simulink model "BlockTest"  (R2017b)
settings: Solver=FixedStepAuto  StartTime=0.0  StopTime=inf  FixedStep=.005  RelTol=1e-3  EnableMultiTasking=on
libraries: arduinolib x2, RASPlib x1, simulink x1
settings Model: SimulationMode=external  ExtModeTrigDuration=2  Creator=nguye  LastModifiedBy=nguye
settings OptimizationCC: PassReuseOutputArgsAs=Individual arguments  MaxStackSize=64
settings DebuggingCC: ParameterTunabilityLossMsg=error
settings HardwareCC: ProdBitPerInt=16  ProdBitPerPointer=16  ProdBitPerSizeT=16  ProdBitPerPtrDiffT=16  ProdLargestAtomicFloat=None  ProdWordSize=8  ProdHWDeviceType=Atmel->AVR
settings SFSimCC: MATLABDynamicMemAlloc=off
settings RTWCC: SystemTargetFile=ert.tlc  HardwareBoard=Arduino Mega 2560  TLCOptions=-aInlineSetEventsForThisBaseRateFcn=TLC_FALSE -aSuppressMultiTaskScheduler=TLC_FALSE -aRateBasedStepFcn=1  TemplateMakefile=ert_default_tmf  GenerateReport=on  Toolchain=Arduino AVR  BuildConfiguration=Faster Runs  IncludeHyperlinkInReport=on  LaunchReport=on  GenerateTraceInfo=on  GenerateTraceReport=on  GenerateTraceReportSl=on  GenerateTraceReportSf=on  GenerateTraceReportEml=on
settings CodeAppCC: ForceParamTrailComments=on  IgnoreCustomStorageClasses=off  OperatorAnnotations=on  SimulinkDataObjDesc=on  SFDataObjDesc=on  InsertBlockDesc=on
settings ERTTargetCC: SupportContinuousTime=on  SupportVariableSizeSignals=on  ExtMode=on  ExtModeMexArgs='127.0.0.1' 0 17725

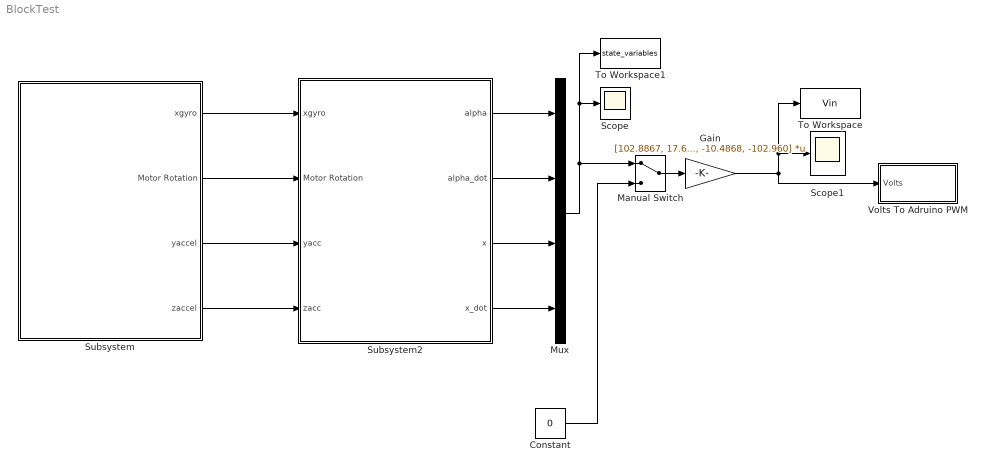
== system BlockTest ==
  Constant : Constant  Value=0
  Gain : Gain  Gain=[102.8867, 17.6796, -10.4868, -102.960]  Multiplication=Matrix(K*u)
  Manual Switch : ManualSwitch
  Mux : Mux
  Scope : Scope
  Scope1 : Scope
  Subsystem : Subsystem
  Subsystem2 : Subsystem
  To Workspace : ToWorkspace  VariableName=Vin  SaveFormat=Timeseries  SampleTime=-1
  To Workspace1 : ToWorkspace  VariableName=state_variables  SampleTime=-1
  Volts To Adruino PWM : Subsystem
  wires:
  Subsystem/1(xgyro) -> Subsystem2/1(xgyro)
  Subsystem/2(Motor Rotation) -> Subsystem2/2(Motor Rotation)
  Mux/1 -> To Workspace1/1, Scope/1, Manual Switch/1
  Manual Switch/1 -> Gain/1
  Constant/1 -> Manual Switch/2
  Gain/1 -> Volts To Adruino PWM/1(Volts), To Workspace/1, Scope1/1
  Subsystem/3(yaccel) -> Subsystem2/3(yacc)
  Subsystem/4(zaccel) -> Subsystem2/4(zacc)
  Subsystem2/4(x_dot) -> Mux/4
  Subsystem2/3(x) -> Mux/3
  Subsystem2/2(alpha_dot) -> Mux/2
  Subsystem2/1(alpha) -> Mux/1

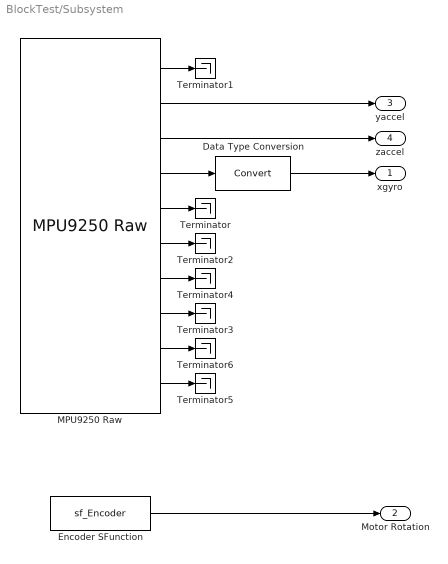
== system BlockTest/Subsystem ==
  Data Type Conversion : DataTypeConversion
  Encoder SFunction : S-Function  InitFcn=try, set_param(gcb,'FunctionName','sf_Encoder'), end  FunctionName=sf_Encoder  Parameters=uint8(0),uint8(18),uint8(19)  SFunctionModules=sf_Encoder_wrapper  SFunctionDeploymentMode=off  EnableBusSupport=off  mask(S-Function Builder){}
      mask init:
      | val = [[.9  0.75 0.75 1 1 .9 .9 1]',[1 1 0.75 0.75 .9 .9 1 .9]'];try , sys = get_param(gcb,'SfunBuilderFcnName');if isempty(sys), sys = get_param(gcb,'FunctionName'); end,catch, sys = get_param(gcb,'FunctionName'); end
      settings: CopyFcn=set_param(gcbh,'LinkStatus','none')  PreSaveFcn=try, set_param(gcb,'FunctionName','sf_Encoder'), end  OpenFcn=sfunctionwizard(gcbh)
      mask Display: plot(val(:,1),val(:,2)),disp(sys), port_label('output',1,'pos')
  MPU9250 Raw : RASPlib/MPU9250 Raw  SimulateUsing=Code generation
      settings: SourceProductName=Rensselaer Arduino Support Package
  Terminator{,1..6} (7 alike) : Terminator
  xgyro : Outport
  Motor Rotation : Outport  Port=2
  yaccel : Outport  Port=3
  zaccel : Outport  Port=4
  wires:
  Encoder SFunction/1 -> Motor Rotation/1
  MPU9250 Raw/4 -> Data Type Conversion/1
  MPU9250 Raw/2 -> yaccel/1
  MPU9250 Raw/3 -> zaccel/1
  MPU9250 Raw/1 -> Terminator1/1
  MPU9250 Raw/5 -> Terminator/1
  MPU9250 Raw/6 -> Terminator2/1
  MPU9250 Raw/7 -> Terminator4/1
  MPU9250 Raw/8 -> Terminator3/1
  MPU9250 Raw/9 -> Terminator6/1
  MPU9250 Raw/10 -> Terminator5/1
  Data Type Conversion/1 -> xgyro/1

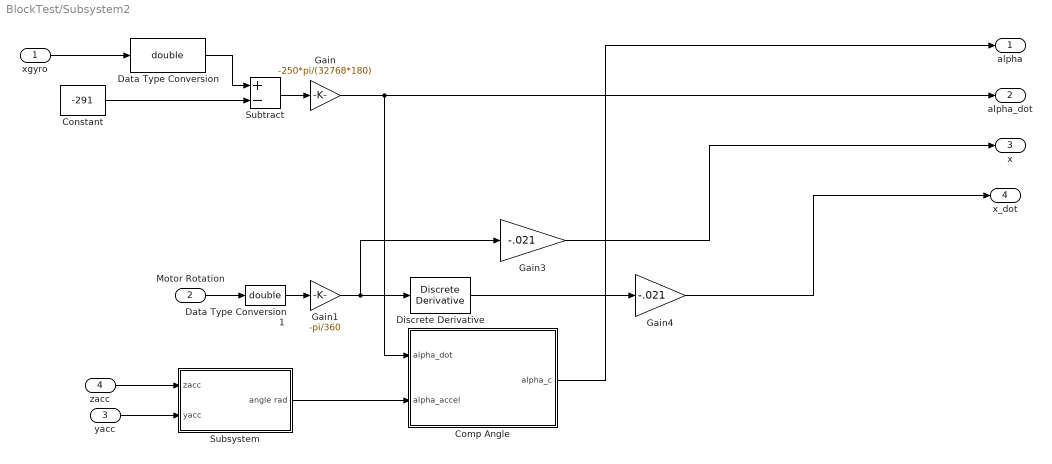
== system BlockTest/Subsystem2 ==
  xgyro : Inport
  Motor Rotation : Inport  Port=2
  yacc : Inport  Port=3
  zacc : Inport  Port=4
  Comp Angle : Subsystem
  Constant : Constant  Value=-291
  Data Type Conversion : DataTypeConversion  OutDataTypeStr=double
  Data Type Conversion1 : DataTypeConversion  OutDataTypeStr=double
  Discrete Derivative : simulink/Discrete/Discrete Derivative  gainval=1.0  ICPrevScaledInput=0.0  InputProcessing=Inherited  OutMin=[]  OutMax=[]  OutDataType=fixdt(1, 16)  OutScaling=2^-10  DoSatur=off
  Gain : Gain  Gain=-250*pi/(32768*180)
  Gain1 : Gain  Gain=-pi/360
  Gain3 : Gain  Gain=-.021
  Gain4 : Gain  Gain=-.021
  Subsystem : Subsystem
  Subtract : Sum  Inputs=+-
  alpha : Outport
  alpha_dot : Outport  Port=2
  x : Outport  Port=3
  x_dot : Outport  Port=4
  wires:
  Data Type Conversion/1 -> Subtract/1
  Constant/1 -> Subtract/2
  Subtract/1 -> Gain/1
  xgyro/1 -> Data Type Conversion/1
  Motor Rotation/1 -> Data Type Conversion1/1
  Gain/1 -> alpha_dot/1, Comp Angle/1(alpha_dot)
  Data Type Conversion1/1 -> Gain1/1
  Gain1/1 -> Gain3/1, Discrete Derivative/1
  Discrete Derivative/1 -> Gain4/1
  Subsystem/1(angle rad) -> Comp Angle/2(alpha_accel)
  Comp Angle/1(alpha_c) -> alpha/1
  Gain4/1 -> x_dot/1
  Gain3/1 -> x/1
  zacc/1 -> Subsystem/1(zacc)
  yacc/1 -> Subsystem/2(yacc)

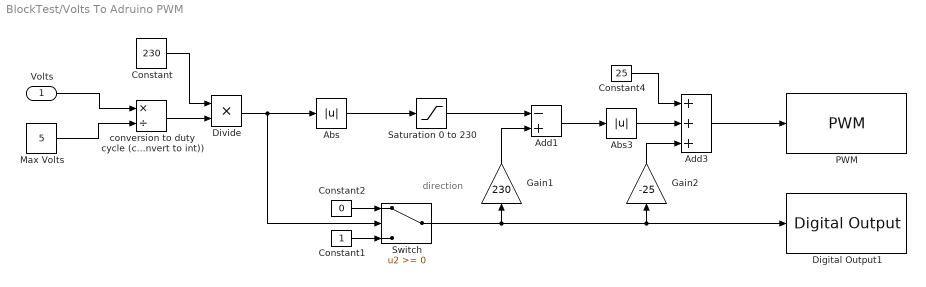
== system BlockTest/Volts To Adruino PWM ==
  note: direction
  Volts : Inport
  Abs : Abs
  Abs3 : Abs
  Add1 : Sum  Inputs=-+
  Add3 : Sum  Inputs=+++
  Constant : Constant  Value=230
  Constant1 : Constant
  Constant2 : Constant  Value=0
  Constant4 : Constant  Value=25
  Digital Output1 : arduinolib/Digital Output  pinNumber=8  blockPlatform=arduino
  Divide : Product  Inputs=**
  Gain1 : Gain  Gain=230
  Gain2 : Gain  Gain=-25
  Max Volts : Constant  Value=5
  PWM : arduinolib/PWM  pinNumber=6  blockPlatform=arduino
  Saturation 0 to 230 : Saturate  UpperLimit=230  LowerLimit=0
  Switch : Switch
  conversion to duty cycle (convert to int)) : Product  Inputs=*/  OutDataTypeStr=double
  wires:
  Abs/1 -> Saturation 0 to 230/1
  Saturation 0 to 230/1 -> Add1/1
  Add1/1 -> Abs3/1
  Gain1/1 -> Add1/2
  Constant1/1 -> Switch/3
  Constant2/1 -> Switch/1
  Switch/1 -> Gain1/1, Gain2/1, Digital Output1/1
  Abs3/1 -> Add3/2
  Add3/1 -> PWM/1
  Constant4/1 -> Add3/1
  Volts/1 -> conversion to duty cycle (convert to int))/1
  Max Volts/1 -> conversion to duty cycle (convert to int))/2
  Divide/1 -> Switch/2, Abs/1
  conversion to duty cycle (convert to int))/1 -> Divide/2
  Constant/1 -> Divide/1
  Gain2/1 -> Add3/3

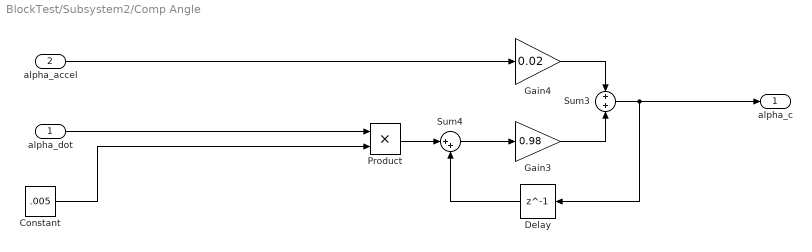
== system BlockTest/Subsystem2/Comp Angle ==
  alpha_dot : Inport
  alpha_accel : Inport  Port=2
  Constant : Constant  Value=.005
  Delay : Delay  DelayLength=1  InitialCondition=0
  Gain3 : Gain  Gain=0.98
  Gain4 : Gain  Gain=0.02
  Product : Product
  Sum3 : Sum
  Sum4 : Sum  Inputs=|++
  alpha_c : Outport
  wires:
  Gain3/1 -> Sum3/2
  Gain4/1 -> Sum3/1
  Sum3/1 -> alpha_c/1, Delay/1
  Sum4/1 -> Gain3/1
  Delay/1 -> Sum4/2
  Product/1 -> Sum4/1
  alpha_accel/1 -> Gain4/1
  alpha_dot/1 -> Product/1
  Constant/1 -> Product/2

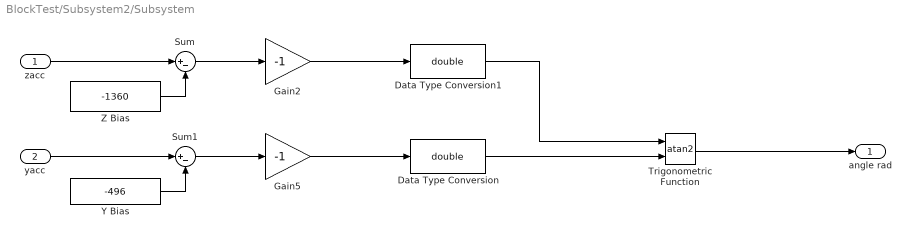
== system BlockTest/Subsystem2/Subsystem ==
  zacc : Inport
  yacc : Inport  Port=2
  Data Type Conversion : DataTypeConversion  OutDataTypeStr=double
  Data Type Conversion1 : DataTypeConversion  OutDataTypeStr=double
  Gain2 : Gain  Gain=-1
  Gain5 : Gain  Gain=-1
  Sum : Sum  Inputs=|+-
  Sum1 : Sum  Inputs=|+-
  Trigonometric Function : Trigonometry  Operator=atan2
  Y Bias : Constant  Value=-496
  Z Bias : Constant  Value=-1360
  angle rad : Outport
  wires:
  Z Bias/1 -> Sum/2
  Y Bias/1 -> Sum1/2
  Trigonometric Function/1 -> angle rad/1
  Data Type Conversion1/1 -> Trigonometric Function/1
  Data Type Conversion/1 -> Trigonometric Function/2
  zacc/1 -> Sum/1
  yacc/1 -> Sum1/1
  Gain2/1 -> Data Type Conversion1/1
  Sum/1 -> Gain2/1
  Sum1/1 -> Gain5/1
  Gain5/1 -> Data Type Conversion/1
